simulink model "mac_df2t_soln"  (Simulink 7.4)
settings: Solver=ode45  StartTime=0.0  StopTime=0.05  RelTol=1e-3
undefined symbols (not defined in the file): Fs, sided, Two, xlfda_numerator
libraries: xbsIndex_r4 x29, dspsnks4 x3, dspobslib x2, xbsCopyrightNotice_r4 x1, dspsrcs4 x1, dsparch3 x1
settings Model: Creator=douangp  LastModifiedBy=douangp
settings DataIOCC: SaveOutput=off  SaveTime=off  SignalLoggingName=sigsOut
settings OptimizationCC: BlockReduction=off  BooleanDataType=off  InitFltsAndDblsToZero=on
settings DebuggingCC: SaveWithParameterizedLinksMsg=none  SignalResolutionControl=TryResolveAllWithWarning  SolverPrmCheckMsg=none  MultiTaskDSMMsg=warning  MultiTaskCondExecSysMsg=none  StrictBusMsg=None
settings HardwareCC: TargetUnknown=on
settings RTWCC: IncludeERTFirstTime=on
settings GRTTargetCC: TargetFcnLib=ansi_tfl_tmw.mat  ModelReferenceCompliant=off  MatFileLogging=off

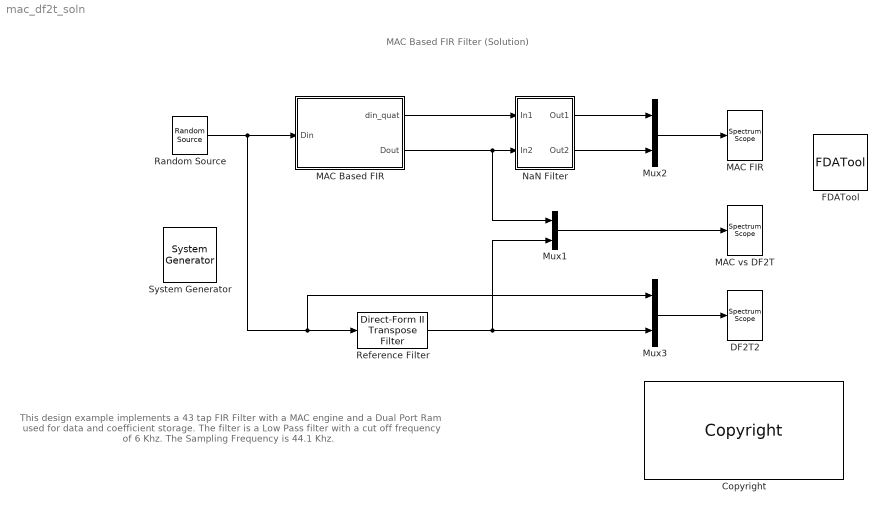
== system mac_df2t_soln ==
  note: This design example implements a 43 tap FIR Filter with a MAC engine
      | and a Dual Port Ram used for data and coefficient storage. The filter is a
      | Low Pass filter with a cut off frequency of 6 Khz. The Sampling Frequency
      | is 44.1 Khz.
  note: MAC Based FIR Filter (Solution)
  " System Generator" : xbsIndex_r4/ System Generator  Tag=genX  SystemSampleTime=-1  xilinxfamily=virtex6  part=xc6vlx240t  speed=-1  package=ff1156  synthesis_tool=XST  clock_wrapper=Clock Enables  directory=./netlist_soln  testbench=off  simulink_period=5.273427200337499e-007  sysclk_period=7  dcm_input_clock_period=100  incr_netlist=off  trim_vbits=According to Block Masks  dbl_ovrd=According to Block Masks  core_generation=According to Block Masks  run_coregen=off  deprecated_control=off  eval_field=0  block_type=sysgen
      settings: block_version=10.1.3
  Copyright : xbsCopyrightNotice_r4/Copyright  copyrighttext="Copyright (c) 2010  by  Xilinx, Inc. All rights reserved.<br><br>This file contains proprietary, confidential information of Xilinx, Inc., is distributed under licensefrom Xilinx, Inc., and may be used, copied and/or disclosed only pursuant to the terms of a valid licenseagreement with Xilinx, Inc. Xilinx hereby grants you a license to use this file solely for design,simulation, implementation and creation of design files limited to Xilinx devices or technologies. Use with non-Xilinx devices or technologies is expressly prohibited and immediately terminates your license unless covered by a separate agreement.<br><br>Xilinx is providing this design, code, or information \"as-is\" solely for use in developing programs and solutions for Xilinx devices, with no obligation on the part of Xilinx to provide support. By providingthis design, code, or information as one possible implementation of this feature, application or standard,Xilinx is making no representation that this implementation is free from any claims of infringement. Youare responsible for obtaining any rights you may require for your implementation. Xilinx expressly disclaimsany warranty whatsoever with respect to the adequacy of the implementation, including but not limited to anywarranties or representations that this implementation is free from claims of infringement, implied warrantiesof merchantability or fitness for a particular purpose.<br><br>Xilinx products are not intended for use in life support appliances, devices, or systems. Use in such applications is expressly prohibited.<br><br>Any modifications that are made to the Source Code are done at the user's sole risk and will be unsupported.<br><br>This copyright and support notice must be retained as part of this text at all times. (c) Copyright 1995-2010 Xilinx, Inc. All rights reserved."  block_type=copyright
      settings: block_version=10.1.3
      settings: infoedit=|
      | Copyright(C) 2008 by  Xilinx, Inc. All rights reserved.<br>
      | <br>
      | This file contains proprietary, confidential information of Xilinx, Inc., is distributed under license
      | from Xilinx, Inc., and may be used, copied and/or disclosed only pursuant to the terms of a valid license
      | agreement with Xilinx, Inc. Xilinx hereby grants you a license to use this file solely for design,
      | simulation, implementation and creation of design files limited to Xilinx devices or technologies. Use
      | with non-Xilinx devices or technologies is expressly prohibited and immediately terminates your license
      | unless covered by a separate agreement.<br>
      | <br>
      | Xilinx is providing this design, code, or information "as-is" solely for use in developing programs and
      | solutions for Xilinx devices, with no obligation on the part of Xilinx to provide support. By providing
      | this design, code, or information as one possible implementation of this feature, application or standard,
      | Xilinx is making no representation that this implementation is free from any claims of infringement. You
      | are responsible for obtaining any rights you may require for your implementation. Xilinx expressly disclaims
      | any warranty whatsoever with respect to the adequacy of the implementation, including but not limited to any
      | warranties or representations that this implementation is free from claims of infringement, implied warranties
      | of merchantability or fitness for a particular purpose.<br>
      | <br>
      | Xilinx products are not intended for use in life support appliances, devices, or systems. Use in such
      | applications is expressly prohibited.<br>
      | <br>
      | Any modifications that are made to the Source Code are done at the user's sole risk and will be unsupported.<br>
      | <br>
      | This copyright and support notice must be retained as part of this text at all times.
      | (c) Copyright 1995-2008 Xilinx, Inc. All rights reserved.
  DF2T2 : dspsnks4/Spectrum Scope  DialogController=dspdialog.SpectrumScope  DialogControllerArgs=DataTag1  SystemSampleTime=-1  ScopeProperties=off  Domain=Frequency  HorizSpan=1  UseBuffer=on  BufferSize=128  Overlap=64  inpFftLenInherit=on  FFTlength=256  numAvg=10  DisplayProperties=off  AxisGrid=on  Memory=off  FrameNumber=on  AxisLegend=on  AxisZoom=off  OpenScopeAtSimStart=on  OpenScopeImmediately=off  FigPos=[621 345 425 130]  AxisProperties=off  XUnits=Hertz  XRange=Two-sided ((-Fs/2...Fs/2])  XDisplay=0  InheritXIncr=off  XIncr=1/44100  XLabel=Samples  XLimit=User-defined  YUnits=dBm  XMax=22050  XMin=0  YLabel=Magnitude, dBm  LineProperties=off  LineColors=[0.1 0.2 0.7]|[0.6 0.2 0.1]|[0.1 0.6 0.1]  wintypeSpecScope=Hann  RsSpecScope=50  betaSpecScope=5  winsampSpecScope=Periodic  XAxisParamsVer=6.9
      settings: YMin=-42.7125  YMax=18
  FDATool : xbsIndex_r4/FDATool  block_type=fdatool
      settings: infoedit=FDATool  block_version=10.1.3
  MAC Based FIR : Subsystem  mask(MAC FIR mask){coef=xlfda_numerator('FDATool'), coef_width=12, coef_binpt=12, data_width=10, data_binpt=8, Fs=44100}
      mask prompts: coef "Filter Coefficients"; coef_width "Coefficient Width"; coef_binpt "Coefficient Binary Point"; data_width "Data Width"; data_binpt "Data Binary Point"; Fs "Sampling Frequency (Hz)"
      mask Display:
      | disp(length(coef))
      | disp('\n\nTaps')
  MAC FIR : dspsnks4/Spectrum Scope  DialogController=dspdialog.SpectrumScope  DialogControllerArgs=DataTag3  SystemSampleTime=-1  ScopeProperties=off  Domain=Frequency  HorizSpan=1  UseBuffer=on  BufferSize=128  Overlap=64  inpFftLenInherit=on  FFTlength=256  numAvg=10  DisplayProperties=off  AxisGrid=on  Memory=off  FrameNumber=on  AxisLegend=on  AxisZoom=off  OpenScopeAtSimStart=on  OpenScopeImmediately=off  FigPos=[620 556 425 164]  AxisProperties=off  XUnits=Hertz  XRange=Two-sided ((-Fs/2...Fs/2])  XDisplay=0  InheritXIncr=off  XIncr=1/44100  XLabel=Samples  XLimit=User-defined  YUnits=dBm  XMax=22050  XMin=0  YLabel=Magnitude, dBm  LineProperties=off  LineColors=[0.1 0.2 0.7]|[0.6 0.2 0.1]|[0.1 0.6 0.1]  wintypeSpecScope=Hann  RsSpecScope=50  betaSpecScope=5  winsampSpecScope=Periodic  XAxisParamsVer=6.9
      settings: YMin=-42.7125  YMax=18
  MAC vs DF2T : dspsnks4/Spectrum Scope  DialogController=dspdialog.SpectrumScope  DialogControllerArgs=DataTag4  SystemSampleTime=-1  ScopeProperties=off  Domain=Frequency  HorizSpan=1  UseBuffer=on  BufferSize=128  Overlap=64  inpFftLenInherit=on  FFTlength=256  numAvg=10  DisplayProperties=off  AxisGrid=on  Memory=off  FrameNumber=on  AxisLegend=on  AxisZoom=off  OpenScopeAtSimStart=on  OpenScopeImmediately=off  FigPos=[66 465 548 257]  AxisProperties=off  XUnits=Hertz  XRange=Two-sided ((-Fs/2...Fs/2])  XDisplay=0  InheritXIncr=off  XIncr=1/44100  XLabel=Samples  XLimit=User-defined  YUnits=dBm  XMax=22050  XMin=0  YLabel=Magnitude, dBm  LineProperties=off  LineColors=[0.1 0.2 0.7]|[0.6 0.2 0.1]|[0.1 0.6 0.1]  wintypeSpecScope=Hann  RsSpecScope=50  betaSpecScope=5  winsampSpecScope=Periodic  XAxisParamsVer=6.9
      settings: YMin=-42.7125  YMax=18
  Mux1 : Mux  Inputs=2
  Mux2 : Mux  Inputs=2
  Mux3 : Mux  Inputs=2
  NaN Filter : Subsystem
  Random Source : dspsrcs4/Random Source  SrcType=Uniform  NormMethod=Ziggurat  CltLength=12  MinVal=-1.99  MaxVal=1.99  MeanVal=0  VarVal=0.5  RepMode=Not repeatable  rawSeed=1  IsInherit=off  SampMode=Discrete  SampTime=1/44100  SampFrame=1  DataType=Double  OutComplex=Real
  Reference Filter : dsparch3/Direct-Form II Transpose Filter  num=xlfda_numerator('FDATool')  den=1  ic=0
  wires:
  Mux1/1 -> MAC vs DF2T/1
  NaN Filter/1(Out1) -> Mux2/1
  NaN Filter/2(Out2) -> Mux2/2
  MAC Based FIR/1(din_quat) -> NaN Filter/1(In1)
  Random Source/1 -> Reference Filter/1, Mux3/1, MAC Based FIR/1(Din)
  Reference Filter/1 -> Mux1/2, Mux3/2
  MAC Based FIR/2(Dout) -> NaN Filter/2(In2), Mux1/1
  Mux2/1 -> MAC FIR/1
  Mux3/1 -> DF2T2/1

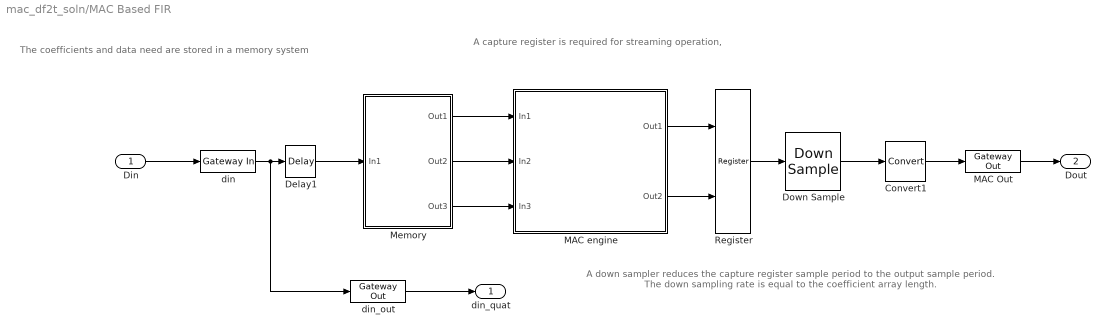
== system mac_df2t_soln/MAC Based FIR ==
  note: A capture register is required for
      | streaming operation,
  note: A down sampler reduces the capture
      | register sample period to the output
      | sample period.
      | The down sampling rate is equal to
      | the coefficient array length.
  note: The coefficients and data need are
      |  stored in a memory system
  Din : Inport  OutDataType=sfix(16)  OutScaling=2^0
  Convert1 : xbsIndex_r4/Convert  arith_type="Signed  (2's comp)"  n_bits=data_width  bin_pt=data_binpt  quantization="Round  (unbiased: +/- Inf)"  overflow=Saturate  en=off  latency=1  dbl_ovrd=off  pipeline=off  block_type=convert
      settings: xl_area=[0, 0, 0, 0, 0, 0, 0]  block_version=VER_STRING_GOES_HERE
  Delay1 : xbsIndex_r4/Delay  en=off  latency=1  dbl_ovrd=off  reg_retiming=off  block_type=delay
      settings: infoedit=Hardware notes: A delay line is a chain, each link of which is an SRL16 followed by a flip-flop. If register retiming is enabled, the delay line is a chain of flip-flops.  xl_area=[0, 0, 0, 0, 0, 0, 0]  block_version=VER_STRING_GOES_HERE
  Down Sample : xbsIndex_r4/Down Sample  sample_ratio=length(coef)  sample_phase="Last Value of Frame  (most efficient)"  en=off  latency=1  dbl_ovrd=off  block_type=dsamp
      settings: xl_area=[0, 0, 0, 0, 0, 0, 0]  block_version=VER_STRING_GOES_HERE
  MAC Out : xbsIndex_r4/Gateway Out  hdl_port=on  timing_constraint=None  locs_specified=off  LOCs={}  block_type=gatewayout
      settings: infoedit="Gateway out block.  Converts Xilinx fixed point inputs into ouputs of type Simulink integer, double, or fixed point.<P><P>Hardware notes:  In hardware these blocks become top level output ports or are discarded, depending on how they are configured."  xl_area=[0, 0, 0, 0, 0, 0, 0]  block_version=VER_STRING_GOES_HERE
  MAC engine : Subsystem
  Memory : Subsystem
  Register : xbsIndex_r4/Register  init=0  rst=off  en=on  dbl_ovrd=off  block_type=register
      settings: xl_area=[0, 0, 0, 0, 0, 0, 0]  block_version=VER_STRING_GOES_HERE
  din : xbsIndex_r4/Gateway In  arith_type="Signed  (2's comp)"  n_bits=data_width  bin_pt=data_binpt  quantization="Round  (unbiased: +/- Inf)"  overflow=Saturate  period=1/Fs  dbl_ovrd=off  timing_constraint=None  locs_specified=off  LOCs={}  hdl_port=on  block_type=gatewayin
      settings: infoedit="Gateway in block.  Converts inputs of type Simulink integer, double and fixed point to  Xilinx fixed point type.<P><P>Hardware notes:  In hardware these blocks become top level input ports."  xl_area=[0, 0, 0, 0, 0, 0, 0]  block_version=VER_STRING_GOES_HERE
  din_out : xbsIndex_r4/Gateway Out  hdl_port=off  timing_constraint=None  locs_specified=off  LOCs={}  block_type=gatewayout
      settings: infoedit="Gateway out block.  Converts Xilinx fixed point inputs into ouputs of type Simulink integer, double, or fixed point.<P><P>Hardware notes:  In hardware these blocks become top level output ports or are discarded, depending on how they are configured."  xl_area=[0, 0, 0, 0, 0, 0, 0]  block_version=VER_STRING_GOES_HERE
  din_quat : Outport  OutDataType=sfix(16)  OutScaling=2^0
  Dout : Outport  Port=2  OutDataType=sfix(16)  OutScaling=2^0
  wires:
  MAC engine/1(Out1) -> Register/1
  Register/1 -> Down Sample/1
  Memory/1(Out1) -> MAC engine/1(In1)
  Memory/2(Out2) -> MAC engine/2(In2)
  Memory/3(Out3) -> MAC engine/3(In3)
  MAC engine/2(Out2) -> Register/2
  din/1 -> Delay1/1, din_out/1
  Delay1/1 -> Memory/1(In1)
  Din/1 -> din/1
  Convert1/1 -> MAC Out/1
  Down Sample/1 -> Convert1/1
  MAC Out/1 -> Dout/1
  din_out/1 -> din_quat/1

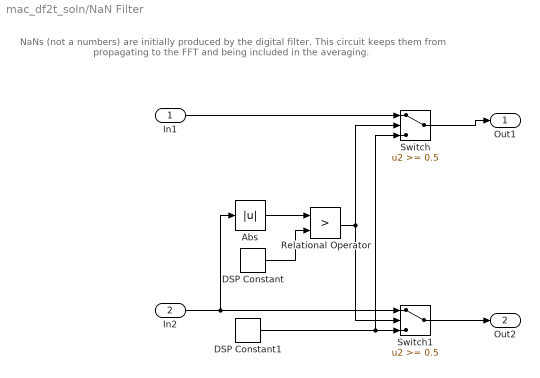
== system mac_df2t_soln/NaN Filter ==
  note: NaNs  (not a numbers) are initially produced by the digital filter.
      | This circuit keeps them from propagating to the FFT and being
      | included in the averaging.
  In1 : Inport  OutDataType=sfix(16)  OutScaling=2^0
  In2 : Inport  Port=2  OutDataType=sfix(16)  OutScaling=2^0
  Abs : Abs  SaturateOnIntegerOverflow=on
  DSP Constant : dspobslib/DSP Constant  SystemSampleTime=-1  Value=-inf  SampleMode=Discrete  discreteOutput=Sample-based  continuousOutput=Sample-based  sampTime=1/22050  framePeriod=1/22050  dataType=Inherit from 'Constant value'  isSigned=on  wordLen=16  udDataType=sfix(16)  fracBitsMode=Best precision  numFracBits=15  InterpretAs1D=off  Ts=1/22050  FramebasedOutput=off
  DSP Constant1 : dspobslib/DSP Constant  SystemSampleTime=-1  Value=0  SampleMode=Discrete  discreteOutput=Sample-based  continuousOutput=Sample-based  sampTime=1/22050  framePeriod=1/22050  dataType=Inherit from 'Constant value'  isSigned=on  wordLen=16  udDataType=sfix(16)  fracBitsMode=Best precision  numFracBits=15  InterpretAs1D=off  Ts=1/22050  FramebasedOutput=off
  Relational Operator : RelationalOperator  Operator=>  InputSameDT=on
  Switch : Switch  Threshold=0.5  SaturateOnIntegerOverflow=on  InputSameDT=on
  Switch1 : Switch  Threshold=0.5  SaturateOnIntegerOverflow=on  InputSameDT=on
  Out1 : Outport  OutDataType=sfix(16)  OutScaling=2^0
  Out2 : Outport  Port=2  OutDataType=sfix(16)  OutScaling=2^0
  wires:
  DSP Constant1/1 -> Switch/3, Switch1/3
  Relational Operator/1 -> Switch1/2, Switch/2
  DSP Constant/1 -> Relational Operator/2
  Abs/1 -> Relational Operator/1
  Switch1/1 -> Out2/1
  Switch/1 -> Out1/1
  In1/1 -> Switch/1
  In2/1 -> Abs/1, Switch1/1

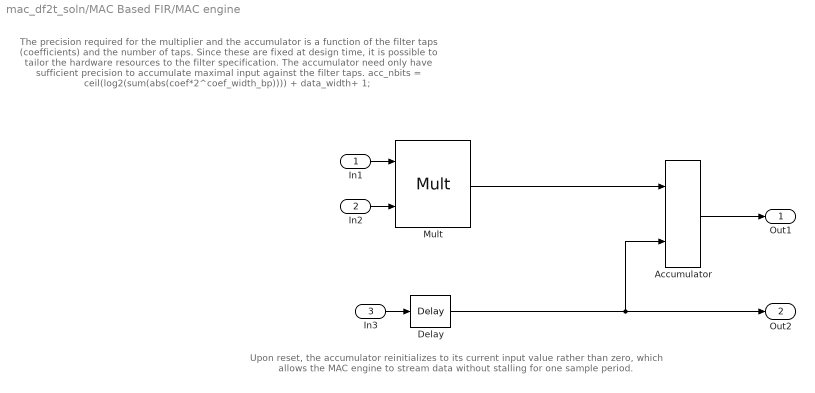
== system mac_df2t_soln/MAC Based FIR/MAC engine ==
  note: The precision required for the multiplier and the accumulator is a
      | function of the filter taps (coefficients) and the number of taps. Since
      | these are fixed at design time, it is possible to tailor the hardware resources
      | to the filter specification.  The accumulator need only have sufficient precision
      | to accumulate maximal input against the filter taps.
      |
      | acc_nbits = ceil(log2(sum(abs(coef*2^coef_width_bp)))) + data_width+ 1;
  note: Upon reset, the accumulator reinitializes to its current input
      | value rather than zero, which allows the MAC engine to stream
      | data without stalling for one sample period.
  In1 : Inport  OutDataType=sfix(16)  OutScaling=2^0
  In2 : Inport  Port=2  OutDataType=sfix(16)  OutScaling=2^0
  In3 : Inport  Port=3  OutDataType=sfix(16)  OutScaling=2^0
  Accumulator : xbsIndex_r4/Accumulator  operation=Add  n_bits=ceil(log2(max(1,sum(abs(coef*2^coef_binpt)))))+data_width +1  overflow=Wrap  scale=1  rst=on  hasbypass=on  en=off  dbl_ovrd=off  use_behavioral_HDL=on  implementation=Fabric  block_type=accum
      settings: infoedit="Adder or subtractor-based accumulator.   Output type and binary point position match the input.<P><P>Hardware notes: When \"Reinitialize with input 'b' on reset\" is selected, the accumulator is forced to run at the system rate even if the input 'b' is running at a slower rate."  xl_area=[0, 0, 0, 0, 0, 0, 0]  block_version=VER_STRING_GOES_HERE
  Delay : xbsIndex_r4/Delay  en=off  latency=3  dbl_ovrd=off  reg_retiming=off  block_type=delay
      settings: infoedit=Hardware notes: A delay line is a chain, each link of which is an SRL16 followed by a flip-flop. If register retiming is enabled, the delay line is a chain of flip-flops.  xl_area=[0, 0, 0, 0, 0, 0, 0]  block_version=VER_STRING_GOES_HERE
  Mult : xbsIndex_r4/Mult  precision=Full  arith_type="Signed  (2's comp)"  n_bits=8  bin_pt=2  quantization=Truncate  overflow=Wrap  en=off  latency=3  dbl_ovrd=off  use_behavioral_HDL=off  opt=Speed  use_embedded=on  optimum_pipeline=off  pipeline=on  use_rpm=on  placement_style=Rectangular shape  block_type=mult
      settings: infoedit=Hardware notes: To use the internal pipeline stage of the dedicated multiplier you must select 'Pipeline to Greatest Extent Possible'.  xl_area=[0, 0, 0, 0, 0, 0, 0]  block_version=VER_STRING_GOES_HERE
  Out1 : Outport  OutDataType=sfix(16)  OutScaling=2^0
  Out2 : Outport  Port=2  OutDataType=sfix(16)  OutScaling=2^0
  wires:
  Mult/1 -> Accumulator/1
  Delay/1 -> Accumulator/2, Out2/1
  In1/1 -> Mult/1
  In2/1 -> Mult/2
  Accumulator/1 -> Out1/1
  In3/1 -> Delay/1

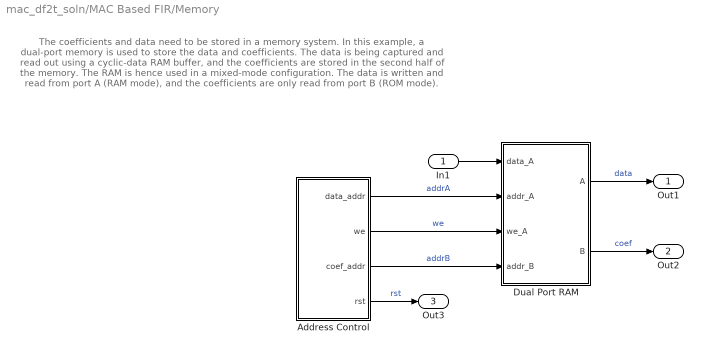
== system mac_df2t_soln/MAC Based FIR/Memory ==
  note: The coefficients and data need to be stored in a memory system.
      | In this example, a dual-port memory is used to store the data and coefficients.
      | The data is being captured and read out using a cyclic-data RAM buffer, and
      | the coefficients are stored in the second half of the memory. The RAM is
      | hence used in a mixed-mode configuration.
      | The data is written and read from port A (RAM mode), and the coefficients are
      | only read from port B (ROM mode).
  In1 : Inport  OutDataType=sfix(16)  OutScaling=2^0
  Address Control : Subsystem
  Dual Port RAM : Subsystem
  Out1 : Outport  OutDataType=sfix(16)  OutScaling=2^0
  Out2 : Outport  Port=2  OutDataType=sfix(16)  OutScaling=2^0
  Out3 : Outport  Port=3  OutDataType=sfix(16)  OutScaling=2^0
  wires:
  Address Control/1(data_addr) -> Dual Port RAM/2(addr_A)  "addrA"
  Address Control/2(we) -> Dual Port RAM/3(we_A)  "we"
  Address Control/3(coef_addr) -> Dual Port RAM/4(addr_B)  "addrB"
  In1/1 -> Dual Port RAM/1(data_A)
  Dual Port RAM/1(A) -> Out1/1  "data"
  Dual Port RAM/2(B) -> Out2/1  "coef"
  Address Control/4(rst) -> Out3/1  "rst"

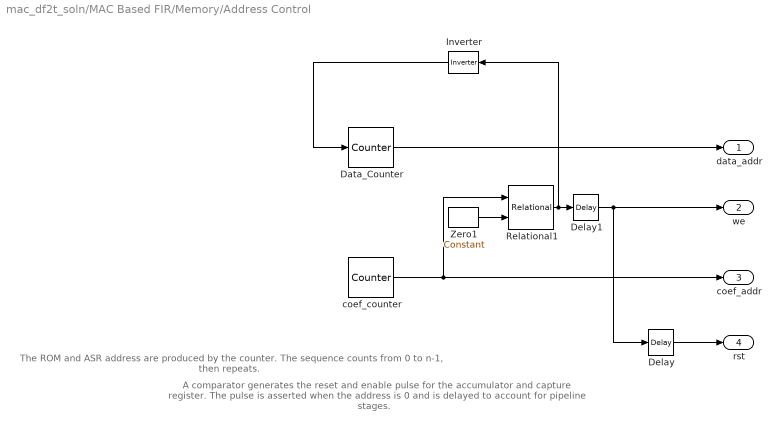
== system mac_df2t_soln/MAC Based FIR/Memory/Address Control ==
  note: The ROM and ASR
      | address are produced
      | by the counter.  The
      | sequence counts from
      | 0 to n-1, then repeats.
  note: A comparator generates
      | the reset and enable
      | pulse for the accumulator
      | and capture register.  The
      | pulse is asserted when
      | the address is 0 and is
      | delayed to account for
      | pipeline stages.
  Data_Counter : xbsIndex_r4/Counter  Priority=5  cnt_type=Count Limited  cnt_to=length(coef)-1  operation=Up  start_count=0  cnt_by_val=1  arith_type=Unsigned  n_bits=ceil(log2(2*length(coef)))  bin_pt=0  load_pin=off  rst=off  en=on  explicit_period=off  period=1  dbl_ovrd=off  use_behavioral_HDL=off  implementation=Fabric  use_rpm=off  block_type=counter
      settings: xl_area=[0, 0, 0, 0, 0, 0, 0]  block_version=VER_STRING_GOES_HERE
  Delay : xbsIndex_r4/Delay  en=off  latency=1  dbl_ovrd=off  reg_retiming=off  block_type=delay
      settings: infoedit=Hardware notes: A delay line is a chain, each link of which is an SRL16 followed by a flip-flop. If register retiming is enabled, the delay line is a chain of flip-flops.  xl_area=[0, 0, 0, 0, 0, 0, 0]  block_version=VER_STRING_GOES_HERE
  Delay1 : xbsIndex_r4/Delay  en=off  latency=1  dbl_ovrd=off  reg_retiming=off  block_type=delay
      settings: infoedit=Hardware notes: A delay line is a chain, each link of which is an SRL16 followed by a flip-flop. If register retiming is enabled, the delay line is a chain of flip-flops.  xl_area=[0, 0, 0, 0, 0, 0, 0]  block_version=VER_STRING_GOES_HERE
  Inverter : xbsIndex_r4/Inverter  en=off  latency=0  dbl_ovrd=off  block_type=inv
      settings: xl_area=[0, 0, 0, 0, 0, 0, 0]  block_version=VER_STRING_GOES_HERE
  Relational1 : xbsIndex_r4/Relational  mode=a=b  en=off  latency=0  dbl_ovrd=off  block_type=relational
      settings: xl_area=[0, 0, 0, 0, 0, 0, 0]  block_version=VER_STRING_GOES_HERE
  Zero1 : xbsIndex_r4/Constant  Priority=5  arith_type=Unsigned  const=2*length(coef)-1  n_bits=ceil(log2(2*length(coef)))  bin_pt=0  explicit_period=off  period=1  equ=P=C  opselect=C  inp2=PCIN>>17  opr=+  inp1=P  carry=CIN  dbl_ovrd=off  block_type=constant
      settings: block_version=VER_STRING_GOES_HERE
  coef_counter : xbsIndex_r4/Counter  Priority=5  cnt_type=Count Limited  cnt_to=2*length(coef)-1  operation=Up  start_count=length(coef)  cnt_by_val=1  arith_type=Unsigned  n_bits=ceil(log2(2*length(coef)))  bin_pt=0  load_pin=off  rst=off  en=off  explicit_period=off  period=1/(Fs*length(coef))  dbl_ovrd=off  use_behavioral_HDL=off  implementation=Fabric  use_rpm=off  block_type=counter
      settings: xl_area=[0, 0, 0, 0, 0, 0, 0]  block_version=VER_STRING_GOES_HERE
  data_addr : Outport  OutDataType=sfix(16)  OutScaling=2^0
  we : Outport  Port=2  OutDataType=sfix(16)  OutScaling=2^0
  coef_addr : Outport  Port=3  OutDataType=sfix(16)  OutScaling=2^0
  rst : Outport  Port=4  OutDataType=sfix(16)  OutScaling=2^0
  wires:
  coef_counter/1 -> coef_addr/1, Relational1/1
  Data_Counter/1 -> data_addr/1
  Zero1/1 -> Relational1/2
  Relational1/1 -> Delay1/1, Inverter/1
  Delay/1 -> rst/1
  Delay1/1 -> Delay/1, we/1
  Inverter/1 -> Data_Counter/1

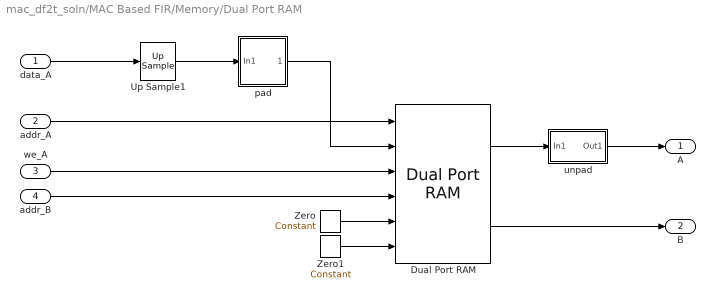
== system mac_df2t_soln/MAC Based FIR/Memory/Dual Port RAM ==
  data_A : Inport  OutDataType=sfix(16)  OutScaling=2^0
  addr_A : Inport  Port=2  OutDataType=sfix(16)  OutScaling=2^0
  we_A : Inport  Port=3  OutDataType=sfix(16)  OutScaling=2^0
  addr_B : Inport  Port=4  OutDataType=sfix(16)  OutScaling=2^0
  Dual Port RAM : xbsIndex_r4/Dual Port RAM  depth=length(coef)*2  initVector=[zeros(1, length(coef)) (coef)]  distributed_mem=Block RAM  init_a=0  init_b=0  rst_a=off  rst_b=off  en_a=off  en_b=off  latency=1  write_mode_A=Read After Write  write_mode_B=Read After Write  dbl_ovrd=off  optimize=Area  use_rpm=off  block_type=dpram
      settings: xl_area=[0, 0, 0, 0, 0, 0, 0]  block_version=VER_STRING_GOES_HERE
  Up Sample1 : xbsIndex_r4/Up Sample  sample_ratio=length(coef)  copy_samples=on  en=off  latency=0  dbl_ovrd=off  block_type=usamp
      settings: infoedit="Up samples input data.  Inserted values  can be zeros or copies of the most recent input sample.<P><P>Hardware notes: No hardware is needed if inserted values are copies of the input sample; otherwise, a mux and single bit flip-flop are used."  xl_area=[0, 0, 0, 0, 0, 0, 0]  block_version=VER_STRING_GOES_HERE
  Zero : xbsIndex_r4/Constant  Priority=5  arith_type=Signed (2's comp)  const=0  n_bits=coef_width  bin_pt=coef_binpt  explicit_period=off  period=1  equ=P=C  opselect=C  inp2=PCIN>>17  opr=+  inp1=P  carry=CIN  dbl_ovrd=off  block_type=constant
      settings: block_version=VER_STRING_GOES_HERE
  Zero1 : xbsIndex_r4/Constant  Priority=5  arith_type=Boolean  const=0  n_bits=1  bin_pt=0  explicit_period=off  period=1  equ=P=C  opselect=C  inp2=PCIN>>17  opr=+  inp1=P  carry=CIN  dbl_ovrd=off  block_type=constant
      settings: block_version=VER_STRING_GOES_HERE
  pad : Subsystem
  unpad : Subsystem
  A : Outport  OutDataType=sfix(16)  OutScaling=2^0
  B : Outport  Port=2  OutDataType=sfix(16)  OutScaling=2^0
  wires:
  Dual Port RAM/2 -> B/1
  Zero/1 -> Dual Port RAM/5
  Zero1/1 -> Dual Port RAM/6
  Dual Port RAM/1 -> unpad/1(In1)
  data_A/1 -> Up Sample1/1
  addr_A/1 -> Dual Port RAM/1
  unpad/1(Out1) -> A/1
  we_A/1 -> Dual Port RAM/3
  addr_B/1 -> Dual Port RAM/4
  pad/1(Out1) -> Dual Port RAM/2
  Up Sample1/1 -> pad/1(In1)

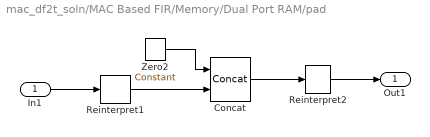
== system mac_df2t_soln/MAC Based FIR/Memory/Dual Port RAM/pad ==
  In1 : Inport  OutDataType=sfix(16)  OutScaling=2^0
  Concat : xbsIndex_r4/Concat  num_inputs=2  dbl_ovrd=off  block_type=concat
      settings: block_version=VER_STRING_GOES_HERE
  Reinterpret1 : xbsIndex_r4/Reinterpret  force_arith_type=on  arith_type=Unsigned  force_bin_pt=on  bin_pt=0  block_type=cast
      settings: infoedit="Changes type of samples without altering their binary representation.<P><P>Hardware notes: In hardware this block costs nothing.<P><P>Example:  Suppose the input is 6 bits wide, signed, with 2 fractional bits, and the output is forced to unsigned with 0 fractional bits.  Then an input of -2.0 (1110.00 in binary 2's complement) becomes an output of 56 (111000 in binary)."  block_version=VER_STRING_GOES_HERE
  Reinterpret2 : xbsIndex_r4/Reinterpret  force_arith_type=on  arith_type="Signed  (2's comp)"  force_bin_pt=on  bin_pt=coef_binpt  block_type=cast
      settings: infoedit="Changes type of samples without altering their binary representation.<P><P>Hardware notes: In hardware this block costs nothing.<P><P>Example:  Suppose the input is 6 bits wide, signed, with 2 fractional bits, and the output is forced to unsigned with 0 fractional bits.  Then an input of -2.0 (1110.00 in binary 2's complement) becomes an output of 56 (111000 in binary)."  block_version=VER_STRING_GOES_HERE
  Zero2 : xbsIndex_r4/Constant  Priority=5  arith_type=Unsigned  const=0  n_bits=coef_width-data_width  bin_pt=0  explicit_period=off  period=1  equ=P=C  opselect=C  inp2=PCIN>>17  opr=+  inp1=P  carry=CIN  dbl_ovrd=off  block_type=constant
      settings: block_version=VER_STRING_GOES_HERE
  Out1 : Outport  OutDataType=sfix(16)  OutScaling=2^0
  wires:
  Zero2/1 -> Concat/1
  Reinterpret1/1 -> Concat/2
  Concat/1 -> Reinterpret2/1
  In1/1 -> Reinterpret1/1
  Reinterpret2/1 -> Out1/1

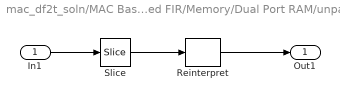
== system mac_df2t_soln/MAC Based FIR/Memory/Dual Port RAM/unpad ==
  In1 : Inport  OutDataType=sfix(16)  OutScaling=2^0
  Reinterpret : xbsIndex_r4/Reinterpret  force_arith_type=on  arith_type="Signed  (2's comp)"  force_bin_pt=on  bin_pt=data_binpt  block_type=cast
      settings: infoedit="Changes type of samples without altering their binary representation.<P><P>Hardware notes: In hardware this block costs nothing.<P><P>Example:  Suppose the input is 6 bits wide, signed, with 2 fractional bits, and the output is forced to unsigned with 0 fractional bits.  Then an input of -2.0 (1110.00 in binary 2's complement) becomes an output of 56 (111000 in binary)."  block_version=VER_STRING_GOES_HERE
  Slice : xbsIndex_r4/Slice  nbits=data_width  boolean_output=off  mode=Lower Bit Location + Width  bit1=0  base1=MSB of Input  bit0=0  base0=LSB of Input  dbl_ovrd=off  block_type=slice
      settings: infoedit="Extracts a given range of bits from each input sample and presents it at the output.  The output type is ordinarily unsigned with binary point at zero, but can be Boolean when the slice is one bit wide.<P><P>Hardware notes: In hardware this block costs nothing."  block_version=VER_STRING_GOES_HERE
  Out1 : Outport  OutDataType=sfix(16)  OutScaling=2^0
  wires:
  Slice/1 -> Reinterpret/1
  In1/1 -> Slice/1
  Reinterpret/1 -> Out1/1
